simulink model "Arrays2"  (Simulink 8.7)
settings: Solver=FixedStepDiscrete  StartTime=0.0  StopTime=10000.0  RelTol=1e-3
settings Model: Creator=scaife  LastModifiedBy=hamza  ExtModeAutoUpdateStatusClock=off
settings DataIOCC: SignalLoggingSaveFormat=ModelDataLogs  SignalLoggingName=sigsOut
settings DebuggingCC: SaveWithParameterizedLinksMsg=none  SignalResolutionControl=TryResolveAllWithWarning  MultiTaskDSMMsg=warning  MultiTaskCondExecSysMsg=none  StrictBusMsg=None
settings HardwareCC: TargetUnknown=on
settings SFSimCC: SimParseCustomCode=off
settings GRTTargetCC: GeneratePreprocessorConditionals=Use local settings  CombineOutputUpdateFcns=off  GRTInterface=on

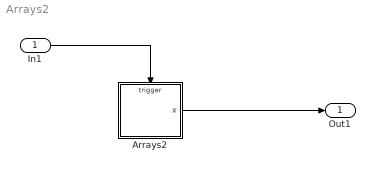
== system Arrays2 ==
  In1 : Inport
  Arrays2 : Stateflow chart  TreatAsAtomicUnit=on
  Out1 : Outport
  wires:
  In1/1 -> Arrays2/Trigger
  Arrays2/1(x) -> Out1/1

== stateflow chart Arrays2 ==
  state A/
    en:x[1][1]++
    x[2][1]--
  state B/
    en:x[1][2]++
    x[2][2]--
  state C/
    en:x[1][3]++
    x[2][3]--
  (default) -> A
  A -> B : E
  C -> A : E
  B -> C : E
  data: x output double size=[2 3] [0..100] =1
  events: E input RISING_EDGE_EVENT
